simulink model "dead_zone_assignment"  (R2020a)
settings: Solver=VariableStepAuto  StartTime=0.0  StopTime=10.0  RelTol=1e-3
libraries: simulink x2
settings Model: Creator=Ujwal  LastModifiedBy=Ujwal

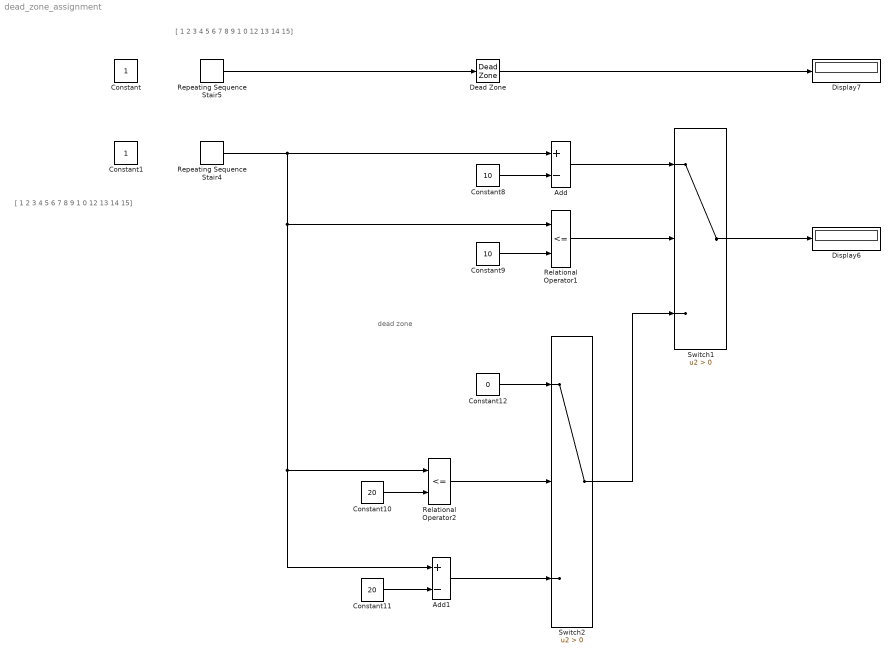
== system dead_zone_assignment ==
  note: [ 1 2 3 4 5 6 7 8 9 1 0 12 13 14 15]
  note: dead zone
  note: [ 1 2 3 4 5 6 7 8 9 1 0 12 13 14 15]
  Add : Sum  Inputs=+-
  Add1 : Sum  Inputs=+-
  Constant : Constant
  Constant1 : Constant
  Constant10 : Constant  Value=20
  Constant11 : Constant  Value=20
  Constant12 : Constant  Value=0
  Constant8 : Constant  Value=10
  Constant9 : Constant  Value=10
  Dead Zone : DeadZone  LowerValue=10  UpperValue=20  SaturateOnIntegerOverflow=on
  Display6 : Display
  Display7 : Display
  Relational Operator1 : RelationalOperator  Operator=<=  OutDataTypeStr=boolean  RndMeth=Simplest
  Relational Operator2 : RelationalOperator  Operator=<=  OutDataTypeStr=boolean  RndMeth=Simplest
  Repeating Sequence Stair4 : simulink/Sources/Repeating Sequence Stair  OutValues="[ 1 2 3 4 5 6 7 8 9 10 12 13  14 15 16 17 18 19 20 21 22 23 24 25]"  tsamp=-1  OutMin=[]  OutMax=[]  OutDataTypeStr=double  OutputDataTypeScalingMode=double  OutDataType=fixdt(0,8)  ConRadixGroup=Best Precision: Vector-wise  OutScaling=2^-12
  Repeating Sequence Stair5 : simulink/Sources/Repeating Sequence Stair  OutValues="[ 1 2 3 4 5 6 7 8 9 10 12 13  14 15 16 17 18 19 20 21 22 23 24 25]"  tsamp=-1  OutMin=[]  OutMax=[]  OutDataTypeStr=double  OutputDataTypeScalingMode=double  OutDataType=fixdt(0,8)  ConRadixGroup=Best Precision: Vector-wise  OutScaling=2^-12
  Switch1 : Switch  Criteria=u2 > Threshold
  Switch2 : Switch  Criteria=u2 > Threshold
  wires:
  Relational Operator2/1 -> Switch2/2
  Dead Zone/1 -> Display7/1
  Add1/1 -> Switch2/3
  Constant8/1 -> Add/2
  Switch1/1 -> Display6/1
  Constant10/1 -> Relational Operator2/2
  Repeating Sequence Stair5/1 -> Dead Zone/1
  Constant12/1 -> Switch2/1
  Constant11/1 -> Add1/2
  Add/1 -> Switch1/1
  Repeating Sequence Stair4/1 -> Add1/1, Relational Operator2/1, Relational Operator1/1, Add/1
  Switch2/1 -> Switch1/3
  Constant9/1 -> Relational Operator1/2
  Relational Operator1/1 -> Switch1/2
